simulink model "task2mPAM_22_110107589"  (R2023b)
settings: Solver=FixedStepAuto  StartTime=0.0  StopTime=8*8-1  RelTol=1e-3
libraries: commchan3 x1, dspstat3 x1, dspsrcs4 x1, dspsigops x1
settings Model: LastModifiedBy=gowrav -local
settings OptimizationCC: ReuseModelBlockBuffer=off

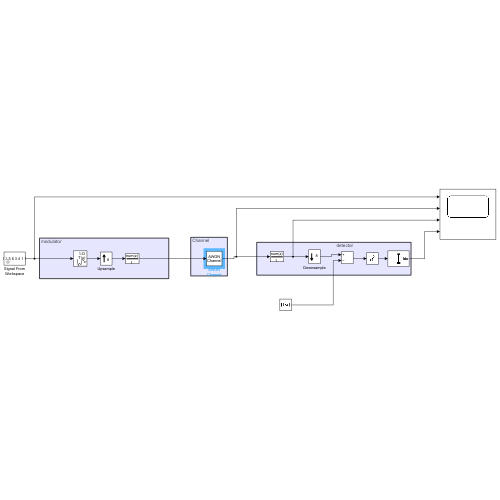
[thumbnail: Simulink's stored preview of the top-level diagram]
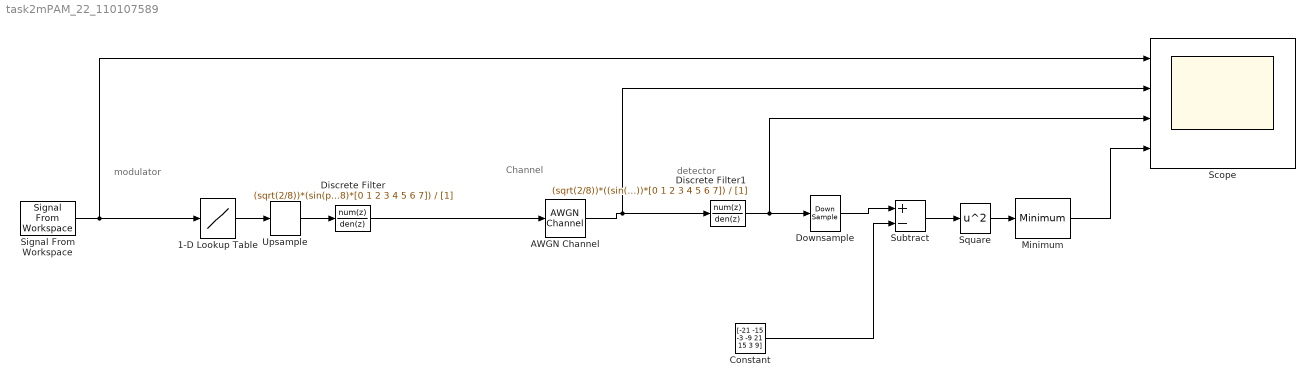
== system task2mPAM_22_110107589 ==
  note: detector
  note: Channel
  note: modulator
  1-D Lookup Table : Lookup_n-D  NumberOfTableDimensions=1  BreakpointsForDimension1=[0:7]  Table=[--21 -15 -3 -9 21 15 3 9 ]  InternalRulePriority=Speed  RndMeth=Simplest
  AWGN Channel : commchan3/AWGN Channel  LegacyMode=on  NoiseMethod="Signal to noise ratio  (SNR)"  noiseMode="Signal to noise ratio  (Es/No)"  EbNo=10  EsNo=40  SNR=10  BitsPerSymbol=1  SignalPower=1  SamplesPerSymbol=1  SymbolPeriod=(1.000000e+00 * 1)  VarianceSource=Parameter  Variance=1  RandomStream=Global stream  Seed=110107589  SimulateUsing=Code generation
  Constant : Constant  Value=[-21 -15 -3 -9 21 15 3 9]
  Discrete Filter : DiscreteFilter  Numerator=(sqrt(2/8))*(sin(pi/8)*[0 1 2 3 4 5 6 7])  Denominator=[1]
  Discrete Filter1 : DiscreteFilter  Numerator=(sqrt(2/8))*((sin(pi/8))*[0 1 2 3 4 5 6 7])  Denominator=[1]
  Downsample : DownSample  N=8  RateOptions=Allow multirate processing
  Minimum : dspstat3/Minimum  operation=minimum  fcn=Index  indexBase=Zero  operateOver=Each column  Dimension=1  InputProcessing=Columns as channels (frame based)  reset=None  roiEnable=off  roiType=Rectangles  roiPortion=Entire ROI  roiOutput=Individual statistics for each ROI  roiFlag=off  roundingMode=Floor  overflowMode=off
  Scope : Scope  NumInputPorts=4
  Signal From Workspace : dspsrcs4/Signal From Workspace  X=[0 2 5 6 3 4 1 7]  Ts=8  nsamps=1  OutputAfterFinalValue=Setting to zero  ignoreOrWarnInputAndFrameLengths=off  OutputFrames=off
  Square : Math  Operator=square
  Subtract : Sum  Inputs=+-
  Upsample : dspsigops/Upsample  FactorSource=Dialog parameter  N=8  Nmax=16  phase=0  RateOptions=Allow multirate processing  ic=0  mode=Unused parameter value
  wires:
  1-D Lookup Table/1 -> Upsample/1
  Upsample/1 -> Discrete Filter/1
  Discrete Filter/1 -> AWGN Channel/1
  AWGN Channel/1 -> Scope/2, Discrete Filter1/1
  Discrete Filter1/1 -> Scope/3, Downsample/1
  Downsample/1 -> Subtract/1
  Constant/1 -> Subtract/2
  Subtract/1 -> Square/1
  Square/1 -> Minimum/1
  Minimum/1 -> Scope/4
  Signal From Workspace/1 -> Scope/1, 1-D Lookup Table/1
